simulink library "aerosimlib"  (Simulink 5.0)
values from neighbouring files (symbols this model uses):
  stdatm = [0 100 200 300 400 500 600 700 800 900 1000 1100 ... (4305 elements, 861x5)]    [stdatm.mat]
undefined symbols (not defined in the file or in its folder): AlphaBnd, b, BetaBnd, CDda, CDde, CDdf, CDdr, CDM, CDmin, CGempty, CGgross, CL0, CLa, CLalphadot, Clbeta, Clda, CLde, CLdf, Cldr, CLM, CLmind, Clp, CLq, Clr, Cm0, Cma, Cmalphadot, Cmde, Cmdf, CmM, Cmq, Cnbeta, Cnda, Cndr, Cnp, Cnr, CP, CT, CYbeta, CYda, CYdr, CYp, CYr, Displacement, dmy, Engine, EulerIni, FuelFlow, FuelIni, J, Jempty, Jeng, Jgross, Jprop, MAC, MAP, MAPLim, MassIni, MaxPower, mempty ... (+25)
libraries: aerosimlib x350, simulink3 x41
(part 2 of 10)

== system aerosimlib/Math ==
  2pi Bound : Subsystem
      mask Type: 2pi bound
      mask Description: Bounds the input angle to [0, 2pi]. When 0 bound is exceeded the output wraps back to 2pi; when the 2pi bound is exceeded the output wraps back to 0.
      mask Help:
      | Bounds the input angle to [0, 2pi]. When 0 bound is exceeded the output wraps back to 2pi; when the 2pi bound is exceeded the output wraps back to 0.
      | <P><B>Input:</B> any angle in radians, from -Inf to Inf;</P>
      | <P><B>Output:</B> an angle in radians between zero and 2pi.</P>
  Cross Product : Subsystem
      mask Type: Cross product
      mask Description: Computes the cross product of two vectors.
      mask Help:
      | The block computes the cross product of two three-dimensional vectors.
      | <P><B>Inputs:</B> two 3x1 vectors;</P>
      | <P><B>Output:</B> the 3x1 cross product vector.</P>
  Non-zero Sign : Subsystem
      mask Type: Non-zero sign
      mask Description: Sign function outputs 1 for input greater than or equal to 0, and -1 otherwise.
      mask Help: Sign function outputs 1 for input greater than or equal to 0, and -1 otherwise.
  Normalization : Subsystem
      mask Type: Vector normalization
      mask Description: Normalize a vector, e = v/|v|.
      mask Help:
      | The block normalizes the input vector.
      | <P><B>Input:</B> the nx1 vector;</P>
      | <P><B>Output:</B> the nx1 unit vector.</P>
  Vector norm : Subsystem
      mask Type: Vector norm-2
      mask Description: Compute the 2-norm (magnitude) of a vector, |v| = sqrt(v'v).
      mask Help:
      | The block compute the 2-norm (or magnitude) of a vector.
      | <P><B>Input:</B> nx1 vector;</P>
      | <P><B>Output:</B> scalar magnitude.</P>
  Zero Offset : Subsystem  mask(Zero offset){tol=10^-6}
      mask prompts: tol "Tolerance"
      mask help: This block outputs a value equal to the tolerance specified in the block parameters if the input falls within a sphere with this tolerance as radius and center in the origin. Otherwise, the output equals the input.
      mask Help: This block outputs a value equal to the tolerance specified in the block parameters if the input falls within a sphere with this tolerance as radius and center in the origin. Otherwise, the output equals the input.
  pi Bound : Subsystem
      mask Type: pi bound
      mask Description: Bounds the input angle to [-pi, pi]. When -pi bound is exceeded the output wraps back to pi; when the pi bound is exceeded the output wraps back to -pi.
      mask Help:
      | Bounds the input angle to [-pi, pi]. When -pi bound is exceeded the output wraps back to pi; when the pi bound is exceeded the output wraps back to -pi.
      | <P><B>Input:</B> any angle in radians, from -Inf to Inf;</P>
      | <P><B>Output:</B> an angle in radians between -pi and pi.</P>

== system aerosimlib/Pilot Interface ==
  CH F-16 Combat Stick : Subsystem  mask(CH F-16 Combat Stick){joyid=1, tsamp=0.02}
      mask prompts: joyid "Joystick ID:"; tsamp "Sample time:"
      mask help: Joystick interface for F-16 Combat Stick by CH Products.
      mask Help:
      | The block provides interface for the F-16 Combat Stick by CH Products.
      | <P><B>Outputs:</B>
      | <LI>Horiz axis = the current joystick position on the horizontal axis</LI>
      | <LI>Vert axis = the current joystick position on the vertical axis</LI>
      | <LI>Throttle axis = the current position of the throttle wheel</LI>
      | <LI>POV = the current state of the joystick hat switch (0=center, 1=up, -1=down, 2=right, -2=left)</LI>
      | <LI>Button 1-9 = the current states of the 9 available buttons</LI>
      | </P>
      | <P><B>Parameters:</B>
      | <LI>Joystick id = the identifier is used to differentiate between multiple joysticks, and it can be set to 1 or 2.</LI>
      | <LI>Sample time = the time interval at which the joystick data is sampled</LI>
      | </P>
  FS Interface : Subsystem  mask(FS interface){tsamp=0.2}
      mask prompts: tsamp "Sample time:"
      mask help: Microsoft Flight Simulator Interface that provides a visual output of the aircraft position and attitude.
      mask Help:
      | The block provides position and attitude information to Microsoft Flight Simulator for visual output of the aircraft behavior. The data transfer is based on Inter-Process Communication using FSUIPC module.
      | <P><B>Inputs:</B>
      | <LI> the 3x1 vector of geographic position;</LI>
      | <LI> the 3x1 vector of Euler angles;</LI>
      | <LI> scalar number representing airspeed.</LI></P>
  FlightGear Interface : Subsystem  mask(FlightGear 0.9.2 interface){hostname='localhost', port=5500, tsamp=0.02}
      mask prompts: hostname "Host name:"; tsamp "Sample time:"
      mask help:
      | FlightGear Flight Simulator Interface that provides a visual output of the aircraft position and attitude.
      | This driver can be used with FlightGear 0.9.2 only.
      mask Help:
      | The block provides position and attitude information to FlightGear Flight Simulator 0.9.2 for visual output of the aircraft behavior.
      | <P><B>Parameters:</B>
      | <LI>Sample time: the sample time at which data is sent to FlightGear;</LI>
      | <LI>Host name: the name or IP address of the machine on which FlightGear is running.</LI>
      | <LI>Port: the port number on the host machine.</LI>
      | </P>
      | <P><B>Inputs:</B>
      | <LI> the 3x1 vector of geographic position;</LI>
      | <LI> the 3x1 vector of Euler angles;</LI>
      | <LI> scalar number representing airspeed.</LI></P>
  FlightGear 0.9.4  Interface : Subsystem  mask(FlightGear 0.9.4 interface){hostname='localhost', port=5500, tsamp=0.02}
      mask prompts: hostname "Host name:"; tsamp "Sample time:"
      mask help:
      | FlightGear Flight Simulator Interface that provides a visual output of the aircraft position and attitude.
      | This driver can be used with FlightGear 0.9.4 only.
      mask Help:
      | The block provides position and attitude information to FlightGear Flight Simulator 0.9.4 for visual output of the aircraft behavior.
      | <P><B>Parameters:</B>
      | <LI>Sample time: the sample time at which data is sent to FlightGear;</LI>
      | <LI>Host name: the name or IP address of the machine on which FlightGear is running.</LI>
      | <LI>Port: the port number on the host machine.</LI>
      | </P>
      | <P><B>Inputs:</B>
      | <LI>Position =  the 3x1 vector of geographic position in [rad rad m];</LI>
      | <LI>Euler =  the 3x1 vector of Euler angles in radians;</LI>
      | <LI>Airspeed =  scalar number representing airspeed, in m/s;</LI>
      | <LI>VClimb = the climb rate, in m/s;</LI>
      | <LI>AGL = the altitude above ground, in meters;</LI>
      | <LI>VelNED = the 3x1 vector of groundspeed, in m/s;</LI>
      | <LI>Rates = the 3x1 vector of angular rates, in rad/s;</LI>
      | <LI>Acc = the 3x1 vector of body accelerations, in m/s^2;</LI>
      | <LI>Omega = the engine speed,in rad/s;</LI>
      | <LI>FuelFlow = the instananeous fuel flow, in grams per hour;</LI>
      | <LI>OutofFuel = set it to 1 to disable engine noise in FlightGear, otherwise set it to 0;</LI>
      | <LI>Controls = the 7x1 vector of aircraft controls [flap elevator aileron rudder throttle mixture ignition]; the first 4 aerodynamic controls should be normalized to [-1, 1].</LI>
      | </P>
  FlightGear 0.9.6  Interface : Subsystem  mask(FlightGear 0.9.6 interface){hostname='localhost', port=5500, tsamp=0.02}
      mask prompts: hostname "Host name:"; tsamp "Sample time:"
      mask help:
      | FlightGear Flight Simulator Interface that provides a visual output of the aircraft position and attitude.
      | This driver can be used with FlightGear 0.9.6 only.
      mask Help:
      | The block provides position and attitude information to FlightGear Flight Simulator 0.9.6 for visual output of the aircraft behavior.
      | <P><B>Parameters:</B>
      | <LI>Sample time: the sample time at which data is sent to FlightGear;</LI>
      | <LI>Host name: the name or IP address of the machine on which FlightGear is running.</LI>
      | <LI>Port: the port number on the host machine.</LI>
      | </P>
      | <P><B>Inputs:</B>
      | <LI>Position =  the 3x1 vector of geographic position in [rad rad m];</LI>
      | <LI>Euler =  the 3x1 vector of Euler angles in radians;</LI>
      | <LI>Airspeed =  scalar number representing airspeed, in m/s;</LI>
      | <LI>VClimb = the climb rate, in m/s;</LI>
      | <LI>AGL = the altitude above ground, in meters;</LI>
      | <LI>VelNED = the 3x1 vector of groundspeed, in m/s;</LI>
      | <LI>Rates = the 3x1 vector of angular rates, in rad/s;</LI>
      | <LI>Acc = the 3x1 vector of body accelerations, in m/s^2;</LI>
      | <LI>Omega = the engine speed,in rad/s;</LI>
      | <LI>FuelFlow = the instananeous fuel flow, in grams per hour;</LI>
      | <LI>OutofFuel = set it to 1 to disable engine noise in FlightGear, otherwise set it to 0;</LI>
      | <LI>Controls = the 7x1 vector of aircraft controls [flap elevator aileron rudder throttle mixture ignition]; the first 4 aerodynamic controls should be normalized to [-1, 1].</LI>
      | </P>
  FlightGear 0.9.8  Interface : Subsystem  mask(FlightGear 0.9.8 interface){hostname='localhost', port=5500, tsamp=0.02}
      mask prompts: hostname "Host name:"; tsamp "Sample time:"
      mask help:
      | FlightGear Flight Simulator Interface that provides a visual output of the aircraft position and attitude.
      | This driver can be used with FlightGear 0.9.8 only.
      mask Help:
      | The block provides position and attitude information to FlightGear Flight Simulator 0.9.8 for visual output of the aircraft behavior.
      | <P><B>Parameters:</B>
      | <LI>Sample time: the sample time at which data is sent to FlightGear;</LI>
      | <LI>Host name: the name or IP address of the machine on which FlightGear is running.</LI>
      | <LI>Port: the port number on the host machine.</LI>
      | </P>
      | <P><B>Inputs:</B>
      | <LI>Position =  the 3x1 vector of geographic position in [rad rad m];</LI>
      | <LI>Euler =  the 3x1 vector of Euler angles in radians;</LI>
      | <LI>Airspeed =  scalar number representing airspeed, in m/s;</LI>
      | <LI>VClimb = the climb rate, in m/s;</LI>
      | <LI>AGL = the altitude above ground, in meters;</LI>
      | <LI>VelNED = the 3x1 vector of groundspeed, in m/s;</LI>
      | <LI>Rates = the 3x1 vector of angular rates, in rad/s;</LI>
      | <LI>Acc = the 3x1 vector of body accelerations, in m/s^2;</LI>
      | <LI>Omega = the engine speed,in rad/s;</LI>
      | <LI>FuelFlow = the instananeous fuel flow, in grams per hour;</LI>
      | <LI>OutofFuel = set it to 1 to disable engine noise in FlightGear, otherwise set it to 0;</LI>
      | <LI>Controls = the 7x1 vector of aircraft controls [flap elevator aileron rudder throttle mixture ignition]; the first 4 aerodynamic controls should be normalized to [-1, 1].</LI>
      | </P>
  Joystick Interface : Subsystem  mask(Joystick interface){joyid=1, tsamp=0.02}
      mask prompts: joyid "Joystick ID:"; tsamp "Sample time:"
      mask help: Generic Windows joystick interface.
      mask Help:
      | The block provides a generic Windows joystick interface.
      | <P><B>Outputs:</B>
      | <LI>Axes = the 6x1 vector of current joystick position on the 6 available axes</LI>
      | <LI>Buttons = the 32x1 vector of current states of the 32 available buttons (0 or 1)</LI>
      | <LI>POV = the current state of the joystick hat switch (0=center, 1=up, -1=down, 2=right, -2=left)</LI>
      | </P>
      | <P><B>Parameters:</B>
      | <LI>Joystick ID = the identifier can be 1 or 2 and specifies which joystick to read, when the system has two joysticks installed.</LI>
      | <LI>Sample time = the time interval at which the joystick data is sampled</LI>
      | </P>
  R/C Transmitter  Interface : Subsystem  mask(R/C Transmitter Interface){joyid=1, tsamp=0.02}
      mask prompts: joyid "Joystick ID:"; tsamp "Sample time:"
      mask help: The R/C Transmitter Interface can be used with hardware devices that allow the use of R/C radios as Windows-compatible joysticks, such as the RealFlight Transmitter Interface and the Lew Engineering RCJOY.
      mask Help:
      | <P>The R/C Transmitter Interface can be used with hardware devices that allow the use of
      | R/C radios as Windows-compatible joysticks, such as the RealFlight Transmitter
      | Interface and the Lew Engineering RCJOY.</P>
      | <P><B>Outputs:</B>
      | <LI>Ch.1 Aileron = the Channel 1 output (usually aileron or roll cyclic on Futaba radios) normalized to [-1,1]</LI>
      | <LI>Ch.2 Elevator = the Channel 2 output (usually elevator or pitch cyclic on Futaba radios) normalized to [-1,1]</LI>
      | <LI>Ch.3 Throttle = the Channel 3 output (usually throttle/collective on Futaba radios) normalized to [0,1]</LI>
      | <LI>Ch.4 Rudder = the Channel 4 output (usually rudder or tail rotor on Futaba radios) normalize to [-1,1]]</LI>
      | <LI>Ch.5 Gear = the Channel 5 output (usually gear on Futaba radios), discrete 0 or 1</LI>
      | <LI>Ch.6 Flap = the Channel 6 output (usually flap on Futaba radios), discrete 0 or 1</LI>
      | <LI>Ch.7 Aux1 = the Channel 7 output (usually first auxiliary channel), discrete 0 or 1</LI>
      | <LI>Ch.8 Aux2 = the Channel 8 output (usually second auxiliary channel), discrete 0 or 1</LI>
      | </P>
      | <P><B>Parameters:</B>
      | <LI>Joystick id = the identifier is used to differentiate between multiple joysticks, and it can be set to 1 or 2.</LI>
      | <LI>Sample time = the time interval at which the joystick data is sampled</LI>
      | </P>

== system aerosimlib/Propulsion ==
  Fixed-pitch Propeller : Subsystem  mask(Fixed-pitch propeller model){J=J, CT=CT, CP=CP, R=Rprop}
      mask prompts: J "Advance ratio:"; CT "Coefficient of thrust:"; CP "Coefficient of power:"; R "Radius:"
      mask help: Fixed-pitch propeller model using look-up tables of thrust and power coefficients as functions of advance ratio.
      mask Help:
      | The block provides a fixed-pitch propeller model based on look-up tables for thrust and power coefficients as function of the advance ratio.
      | <P><B>Inputs:</B>
      | <LI>Airspeed = the current aircraft airspeed</LI>
      | <LI>rho = the air density at current aircraft altitude</LI>
      | <LI>Omega = the propeller rotation speed</LI>
      | </P>
      | <P><B>Output:</B>
      | <LI>Fprop = the thrust force generated by the propeller (on body x-axis)</LI>
      | <LI>Mprop = the moment generated by the propeller (on body x-axis)</LI>
      | <LI>PropCoeff = the 3x1 vector of propeller coefficients [J CT CP]</LI>
      | </P>
      | <P><B>Parameters:</B>
      | <LI>Advance ratio = the advance ratio vector for interpolation</LI>
      | <LI>Coefficient of thrust = the coefficient of thrust vector for interpolation</LI>
      | <LI>Coefficient of power = the coefficient of power vector for interpolation</LI>
      | <LI>Radius = the propeller radius</LI>
      | </P>
  GA Propulsion System : Subsystem  mask(General-aviation propulsion system){OmegaIni=OmegaIni, RPM=RPM, MAP=MAP, FuelFlow=FuelFlow, Power=Power, Jeng=Jeng, J=J, CT=CT, CP=CP, Rprop=Rprop, Jprop=Jprop, TSL=TSL}
      mask prompts: OmegaIni "Initial engine speed:"; RPM "Engine RPM vector:"; MAP "Engine MAP vector:"; FuelFlow "Engine fuel flow look-up table:"; Power "Engine power look-up table:"; Jeng "Engine moment of inertia:"; J "Propeller advance ratio vector:"; CT "Propeller coefficient of thrust vector:"; CP "Propeller coefficient of power vector:"; Rprop "Propeller radius:"; Jprop "Propeller moment of inertia:"; TSL "Sea-level temperature:"
      mask help: The block models a general aviation propulsion system including a piston engine and a fixed-pitch propeller.
      mask Help:
      | The block provides a general aviation propulsion system using the AeroSim piston engine and fixed-pitch propeller models.
      | <P><B>Inputs:</B>
      | <LI>Control = the 3x1 engine control vector [Throttle Mixture Ignition]</LI>
      | <LI>OutofFuel = the out-of-fuel flag (0 or 1)</LI>
      | <LI>p = the static pressure at current altitude, in Pa</LI>
      | <LI>T = the air temperature at current altitude, in K</LI>
      | <LI>rho = the air density at current altitude, in kg/m^3</LI>
      | <LI>WindAxesVel = the 3x1 vector of body velocities in wind axes [Airspeed Sideslip Angle-of-attack] in [m/s rad rad]</LI>
      | <LI>RST = the integrator reset flag (rising edge)</LI>
      | </P>
      | <P><B>Output:</B>
      | <LI>Fprop = the 3x1 vector of propulsion system forces applied to the airframe, at the propeller hub location</LI>
      | <LI>Mprop = the 3x1 vector of propulsion system moments applied to the airframe</LI>
      | <LI>Omega = the engine shaft rotation speed, in rad/s</LI>
      | <LI>FuelFlow = the mass fuel flow, in kg/s</LI>
      | <LI>EngCoeff = the 5x1 engine coefficient vector [MAP Airflow Fuelflow BSFC Power] in [kPa kg/s kg/s g/(W*hr) W]</LI>
      | <LI>PropCoeff = the 3x1 propeller coefficient vector [J CT CP]</LI>
      | </P>
      | <P><B>Parameters:</B>
      | <LI>Initial engine speed = the initial value for the engine speed, in rad/s</LI>
      | <LI>RPM vector = the engine speed interpolation vector, in rpm</LI>
      | <LI>MAP vector = the manifold air pressure interpolation vector, in kPa</LI>
      | <LI>Fuel flow = the 2-D look-up table for fuel flow, as function of MAP and RPM, in g/hr</LI>
      | <LI>Power = the 2-D look-up table for power, as function of MAP and RPM, in W</LI>
      | <LI>Engine moment of inertia = the moment of inertia of the rotating engine parts (shaft)</LI>
      | <LI>Advance ratio = the advance ratio vector for interpolation</LI>
      | <LI>Coefficient of thrust = the coefficient of thrust vector for interpolation</LI>
      | <LI>Coefficient of power = the coefficient of power vector for interpolation</LI>
      | <LI>Radius = the propeller radius</LI>
      | <LI>Propeller moment of inertia = the moment of inertia of the propeller</LI>
      | <LI>Sea-level temperature = the ambient temperature for which the above engine look-up tables are given</LI>
      | </P>
  Piston Engine : Subsystem  mask(Piston Engine){RPM=RPM, MAP=MAP, fflow=FuelFlow, Power=Power, TSL=TSL}
      mask prompts: RPM "RPM vector:"; MAP "MAP vector:"; fflow "Fuel flow 2-D look-up table:"; Power "Power 2-D look-up table:"; TSL "Sea-level temperature:"
      mask help: The piston engine model computes the engine parameters at current throttle setting, engine rpm, and altitude.
      mask Help:
      | The block provides a piston engine model based on look-up tables for manifold pressure, engine speed (rpm), fuel flow and power.
      | <P><B>Inputs:</B>
      | <LI>Thr = the throttle command (as a fraction of atmospheric pressure)</LI>
      | <LI>Mix = the air to fuel mixture ratio</LI>
      | <LI>Omega = the engine shaft rotation speed</LI>
      | <LI>p = the atmospheric pressure, in Pa</LI>
      | <LI>T = the atmospheric temperature, in K</LI>
      | </P>
      | <P><B>Output:</B>
      | <LI>MAP = the manifold air pressure, in kPa</LI>
      | <LI>AirFlow = the mass air flow, in kg/s</LI>
      | <LI>FuelFlow = the mass fuel flow, in kg/s</LI>
      | <LI>BSFC = the brake-specific fuel consumption, in g/(W*hr)</LI>
      | <LI>Power = the engine power, in W</LI>
      | <LI>Torque = the engine shaft torque, in N*m</LI>
      | </P>
      | <P><B>Parameters:</B>
      | <LI>RPM vector = the engine speed interpolation vector, in rpm</LI>
      | <LI>MAP vector = the manifold air pressure interpolation vector, in kPa</LI>
      | <LI>Fuel flow = the 2-D look-up table for fuel flow, as function of MAP and RPM, in g/hr</LI>
      | <LI>Power = the 2-D look-up table for power, as function of MAP and RPM, in W</LI>
      | <LI>Sea-level temperature = the ambient temperature for which the above engine look-up tables are given</LI>
      | </P>

== system aerosimlib/Sensors ==
  Analog Sensors : Subsystem
  Digital Sensors : Subsystem
  Generic Sensors : Subsystem
  Noise Correlation : Subsystem

== system aerosimlib/Transformations ==
  Body-Inertial DCM From Euler Angles : Subsystem
      mask Type: Body-Inertial DCM
      mask Description: Compute the direction cosine matrix required for inertial-to-body frame transformation.
      mask Help:
      | The block computes the Direction Cosine matrix which is the rotation matrix from inertial to body frame, given the vehicle attitude in Euler angles.
      | <P><B>Input:</B> the 3x1 vector of Euler angles;</P>
      | <P><B>Output:</B> the 3x3 Direction Cosine matrix.</P>
  Body-Inertial DCM From Quaternions : Subsystem
      mask Type: Body-Inertial DCM
      mask Description: Compute the direction cosine matrix required for inertial-to-body frame transformation.
      mask Help:
      | The block computes the Direction Cosine matrix which is the rotation matrix from inertial to body frame, given the Euler-Rodrigues quaternions.
      | <P><B>Input:</B> the 4x1 vector of quaterions;</P>
      | <P><B>Output:</B> the 3x3 Direction Cosine matrix.</P>
  Body-Wind DCM : Subsystem
      mask Type: Body-Wind DCM
      mask Description: Compute the body-axes to wind-axes direction cosine matrix.
      mask Help:
      | The block computes the Direction Cosine matrix that defines the rotation from body to wind axes, given the sideslip angle and the angle-of-attack.
      | <P><B>Input:</B> the 3x1 vector of wind axes velocity components (airspeed, sideslip, angle-of-attack);</P>
      | <P><B>Output:</B> the 3x3 Direction Cosine matrix.</P>
  Body2LTP : Subsystem
      mask Type: Body to LTP
      mask Description: Fast frame transformation from body to local tangential plane (rotation by phi and theta).
  ECEF Position : Subsystem
      mask Type: ECEF Position
      mask Description: Compute ECEF (Earth-centered Earth-fixed) position from LLA (Latitude, Longitude, Altitude) position.
      mask Help:
      | The block computes the coordinates of the vehicle in the Earth-Centered Earth-Fixed frame, given the coordinates in geographic frame and local Earth radii.
      | <P><B>Inputs:</B>
      | <LI>LLA = the 3x1 position vector (Latitude, Longitude, Altitude);</LI>
      | <LI>Rmeridian = local meridian radius of the Earth;</LI>
      | <LI>Rnormal = local normal radius of the Earth;</LI></P>
      | <P><B>Output:</B> the 3x1 vector of ECEF position (X, Y, Z).</P>
  Euler Angles From Quaternions : Subsystem
      mask Type: Euler Angles
      mask Description: Compute Euler angles from Euler-Rodrigues quaternions.
      mask Help:
      | The block computes the three Euler angles (roll, pitch, heading) of the vehicle based on the Euler-Rodrigues quaternions.
      | <P><B>Input:</B> the 4x1 vector of quaternions;</P>
      | <P><B>Output:</B> the 3x1 vector of Euler angles.</P>
  Euler Angles  From DCM : Subsystem
      mask Type: Euler angles from DCM
      mask Description: Compute Euler angles given the Direction Cosine Matrix.
      mask Help:
      | The block extracts the 3 Euler angles (roll, pitch, and heading) from elements of the Direction Cosine matrix.
      | <P><B>Input:</B> a 3x3 Direction Cosine matrix;</P>
      | <P><B>Output:</B> a 3x1 vector with the Euler angles.</P>
  LTP2Body : Subsystem
      mask Type: LTP to Body
      mask Description: Fast frame transformation from local tangential plane to body frame (rotation by phi and theta).
  Quaternions From Euler Angles : Subsystem
      mask Type: Quaternions
      mask Description: Compute quaternions from Euler angles.
      mask Help:
      | The block computes the four quaternions (q0, qx, qy, qz) of the vehicle based on the Euler angles.
      | <P><B>Input:</B> the 3x1 vector of Euler angles.</P>
      | <P><B>Output:</B> the 4x1 vector of quaternions;</P>

== system aerosimlib/Unit Conversion ==
  Angular position : Subsystem
  Angular velocity : Subsystem
  Distance : Subsystem
  Force : Subsystem
  Mass : Subsystem
  Pressure : Subsystem
  Temperature : Subsystem
  Velocity : Subsystem
  Volume : Subsystem

== system aerosimlib/Actuators/D/A Converter ==
  Digital : Inport
  Count size in Volts : Product  Inputs=*/  SaturateOnIntegerOverflow=on  InputSameDT=on
  Max Counts : Constant  Value=2^Bits
  Max Volts : Constant  Value=MaxVolts
  Min Volts : Constant  Value=MinVolts
  Saturation : Saturate  UpperLimit=MaxVolts  LowerLimit=MinVolts
  Sum : Sum  Inputs=|+-  SaturateOnIntegerOverflow=on  InputSameDT=on
  Voltage : Product  SaturateOnIntegerOverflow=on  InputSameDT=on
  Analog : Outport
  wires:
  Digital/1 -> Voltage/1
  Voltage/1 -> Saturation/1
  Max Volts/1 -> Sum/1
  Min Volts/1 -> Sum/2
  Max Counts/1 -> Count size in Volts/2
  Sum/1 -> Count size in Volts/1
  Count size in Volts/1 -> Voltage/2
  Saturation/1 -> Analog/1

== system aerosimlib/Actuators/Simple Actuator (1st-order dynamics) ==
  Input : Inport  PortDimensions=1
  Look-Up Table : Lookup  InputValues=[MinCounts MaxCounts]  OutputValues=[MinAct MaxAct]  SaturateOnIntegerOverflow=on
  Rate Limiter : RateLimiter  RisingSlewLimit=MaxRate  FallingSlewLimit=-MaxRate
  Saturation : Saturate  UpperLimit=MaxCounts  LowerLimit=MinCounts
  Transfer Fcn : TransferFcn  Denominator=[Lag 1]
  Output : Outport
  wires:
  Transfer Fcn/1 -> Output/1
  Rate Limiter/1 -> Transfer Fcn/1
  Saturation/1 -> Look-Up Table/1
  Input/1 -> Saturation/1
  Look-Up Table/1 -> Rate Limiter/1

== system aerosimlib/Actuators/Simple Actuator (2nd-order dynamics) ==
  Input : Inport  PortDimensions=1
  Look-Up Table : Lookup  InputValues=[MinCounts MaxCounts]  OutputValues=[MinAct MaxAct]  SaturateOnIntegerOverflow=on
  Rate Limiter : RateLimiter  RisingSlewLimit=MaxRate  FallingSlewLimit=-MaxRate
  Saturation : Saturate  UpperLimit=MaxCounts  LowerLimit=MinCounts
  Transfer Fcn : TransferFcn  Numerator=[wn^2]  Denominator=[1 2*zeta*wn wn^2]
  Output : Outport
  wires:
  Look-Up Table/1 -> Rate Limiter/1
  Input/1 -> Saturation/1
  Saturation/1 -> Look-Up Table/1
  Rate Limiter/1 -> Transfer Fcn/1
  Transfer Fcn/1 -> Output/1

== system aerosimlib/Aerodynamics/Aerodynamic Force ==
  note: Get aerodynamic forces in
      | wind axes
  note: Get aerodynamic forces
      | in body axes
  CD : Inport  PortDimensions=1
  CY : Inport  Port=2  PortDimensions=1
  CL : Inport  Port=3  PortDimensions=1
  pdyn : Inport  Port=4  PortDimensions=1
  WindAxesVel : Inport  Port=5  PortDimensions=[3 1]
  Body-Wind DCM : aerosimlib/Transformations/Body-Wind DCM
  ChSign : Gain  Gain=-1  SaturateOnIntegerOverflow=on
  ChSign1 : Gain  Gain=-1  SaturateOnIntegerOverflow=on
  DCM' : Math  Operator=transpose
  Mux : Mux  Inputs=3
  Product : Product  Inputs=3  SaturateOnIntegerOverflow=on  InputSameDT=on
  Product1 : Product  Multiplication=Matrix(*)  SaturateOnIntegerOverflow=on  InputSameDT=on
  Wing area : Constant  Value=S
  Faero : Outport
  wires:
  ChSign1/1 -> Mux/3
  ChSign/1 -> Mux/1
  CD/1 -> ChSign/1
  CY/1 -> Mux/2
  CL/1 -> ChSign1/1
  Mux/1 -> Product/1
  pdyn/1 -> Product/2
  Wing area/1 -> Product/3
  WindAxesVel/1 -> Body-Wind DCM/1
  DCM'/1 -> Product1/1
  Body-Wind DCM/1 -> DCM'/1
  Product/1 -> Product1/2
  Product1/1 -> Faero/1

== system aerosimlib/Aerodynamics/Aerodynamic Moment ==
  note: Sources
  note: Compute moments
  note: Output
  Cl : Inport  PortDimensions=1
  Cm : Inport  Port=2  PortDimensions=1
  Cn : Inport  Port=3  PortDimensions=1
  pdyn : Inport  Port=4  PortDimensions=1
  Mux : Mux  Inputs=3
  Pitch : Product  Inputs=4  SaturateOnIntegerOverflow=on  InputSameDT=on
  Roll : Product  Inputs=4  SaturateOnIntegerOverflow=on  InputSameDT=on
  Wing area : Constant  Value=S
  Wing chord : Constant  Value=c
  Wing span : Constant  Value=b
  Yaw : Product  Inputs=4  SaturateOnIntegerOverflow=on  InputSameDT=on
  Maero : Outport
  wires:
  Cl/1 -> Roll/4
  Cm/1 -> Pitch/4
  Cn/1 -> Yaw/4
  pdyn/1 -> Roll/1, Pitch/1, Yaw/1
  Wing area/1 -> Roll/2, Pitch/2, Yaw/2
  Wing chord/1 -> Pitch/3
  Wing span/1 -> Roll/3, Yaw/3
  Roll/1 -> Mux/1
  Mux/1 -> Maero/1
  Pitch/1 -> Mux/2
  Yaw/1 -> Mux/3

== system aerosimlib/Aerodynamics/Drag Coefficient ==
  note: Drag component build-up
  note: Sources
  WindAxesVel : Inport  PortDimensions=[3 1]
  Control : Inport  Port=2  PortDimensions=[4 1]
  CL : Inport  Port=3  PortDimensions=1
  Mach : Inport  Port=4  PortDimensions=1
  Abs{,1..3} (4 alike) : Abs  SaturateOnIntegerOverflow=on
  CD0 : Constant  Value=CD0
  CDM : Gain  Gain=CDM  SaturateOnIntegerOverflow=on
  CDda : Gain  Gain=CDda  SaturateOnIntegerOverflow=on
  CDde : Gain  Gain=CDde  SaturateOnIntegerOverflow=on
  CDdf : Gain  Gain=CDdf  SaturateOnIntegerOverflow=on
  CDdr : Gain  Gain=CDdr  SaturateOnIntegerOverflow=on
  CL min drag : Constant  Value=CL0
  CL^2 : Math  Operator=square
  Demux : Demux
  Demux1 : Demux  Outputs=3
  Induced Drag : Gain  Gain=k  SaturateOnIntegerOverflow=on
  Sum : Sum  Inputs=|+-  SaturateOnIntegerOverflow=on  InputSameDT=on
  Sum2 : Sum  Inputs=+++++++  SaturateOnIntegerOverflow=on  InputSameDT=on
  Terminator : Terminator
  Terminator1 : Terminator
  Terminator2 : Terminator
  CD : Outport
  wires:
  CDM/1 -> Sum2/7
  Mach/1 -> CDM/1
  CL min drag/1 -> Sum/2
  CL/1 -> Sum/1
  Sum/1 -> CL^2/1
  Sum2/1 -> CD/1
  CDdr/1 -> Abs3/1
  CDda/1 -> Abs2/1
  CDde/1 -> Abs1/1
  CDdf/1 -> Abs/1
  Induced Drag/1 -> Sum2/2
  CD0/1 -> Sum2/1
  CL^2/1 -> Induced Drag/1
  Control/1 -> Demux/1
  Demux/4 -> CDdr/1
  Demux/3 -> CDda/1
  Demux/2 -> CDde/1
  Demux/1 -> CDdf/1
  WindAxesVel/1 -> Demux1/1
  Abs/1 -> Sum2/3
  Abs1/1 -> Sum2/4
  Abs2/1 -> Sum2/5
  Abs3/1 -> Sum2/6
  Demux1/1 -> Terminator/1
  Demux1/2 -> Terminator1/1
  Demux1/3 -> Terminator2/1

== system aerosimlib/Aerodynamics/Dynamic Pressure ==
  WindAxesVel : Inport  PortDimensions=[3 1]
  rho : Inport  Port=2  PortDimensions=1
  0.5*rho*Va^2 : Product  SaturateOnIntegerOverflow=on  InputSameDT=on
  Demux : Demux  Outputs=3
  Gain : Gain  Gain=1/2  SaturateOnIntegerOverflow=on
  Terminator : Terminator
  Terminator1 : Terminator
  Va^2 : Math  Operator=square
  pdyn : Outport
  wires:
  rho/1 -> Gain/1
  Demux/3 -> Terminator1/1
  Demux/2 -> Terminator/1
  Demux/1 -> Va^2/1
  WindAxesVel/1 -> Demux/1
  Va^2/1 -> 0.5*rho*Va^2/1
  Gain/1 -> 0.5*rho*Va^2/2
  0.5*rho*Va^2/1 -> pdyn/1

== system aerosimlib/Aerodynamics/Lift Coefficient ==
  note: Lift component build-up
  note: Sources
  WindAxesVel : Inport  PortDimensions=[3 1]
  Control : Inport  Port=2  PortDimensions=[4 1]
  AlphaBetaDot : Inport  Port=3  PortDimensions=[2 1]
  AngularRates : Inport  Port=4  PortDimensions=[3 1]
  Mach : Inport  Port=5  PortDimensions=1
  2 : Gain  Gain=2  SaturateOnIntegerOverflow=on
  CL*c/(2V) : Product  Inputs=**/  SaturateOnIntegerOverflow=on  InputSameDT=on
  CL0 : Constant  Value=CL0
  CLM : Gain  Gain=CLM  SaturateOnIntegerOverflow=on
  CLalpha : Gain  Gain=CLalpha  SaturateOnIntegerOverflow=on
  CLalphadot : Gain  Gain=CLalphadot  SaturateOnIntegerOverflow=on
  CLde : Gain  Gain=CLde  SaturateOnIntegerOverflow=on
  CLdf : Gain  Gain=CLdf  SaturateOnIntegerOverflow=on
  CLq : Gain  Gain=CLq  SaturateOnIntegerOverflow=on
  Demux : Demux
  Demux1 : Demux  Outputs=3
  Demux2 : Demux  Outputs=2
  Demux3 : Demux  Outputs=3
  Sum : Sum  SaturateOnIntegerOverflow=on  InputSameDT=on
  Sum2 : Sum  Inputs=++++++  SaturateOnIntegerOverflow=on  InputSameDT=on
  Terminator{,1..5} (6 alike) : Terminator
  Wing chord : Constant  Value=c
  CL : Outport
  wires:
  CLM/1 -> Sum2/6
  Mach/1 -> CLM/1
  Demux3/3 -> Terminator5/1
  Demux3/2 -> CLq/1
  Demux3/1 -> Terminator4/1
  AngularRates/1 -> Demux3/1
  Sum2/1 -> CL/1
  CL*c/(2V)/1 -> Sum2/5
  CLde/1 -> Sum2/4
  CLdf/1 -> Sum2/3
  CLalpha/1 -> Sum2/2
  CL0/1 -> Sum2/1
  Sum/1 -> CL*c/(2V)/1
  CLalphadot/1 -> Sum/1
  AlphaBetaDot/1 -> Demux2/1
  Demux2/2 -> Terminator3/1
  Demux2/1 -> CLalphadot/1
  Control/1 -> Demux/1
  Demux/4 -> Terminator2/1
  Demux/3 -> Terminator1/1
  Demux/2 -> CLde/1
  Demux/1 -> CLdf/1
  Demux1/3 -> CLalpha/1
  Demux1/2 -> Terminator/1
  Demux1/1 -> 2/1
  CLq/1 -> Sum/2
  Wing chord/1 -> CL*c/(2V)/2
  2/1 -> CL*c/(2V)/3
  WindAxesVel/1 -> Demux1/1

== system aerosimlib/Aerodynamics/Pitch Moment Coefficient ==
  note: Pitch moment component build-up
  note: Sources
  WindAxesVel : Inport  PortDimensions=[3 1]
  Control : Inport  Port=2  PortDimensions=[4 1]
  AlphaBetaDot : Inport  Port=3  PortDimensions=[2 1]
  AngularRates : Inport  Port=4  PortDimensions=[3 1]
  Mach : Inport  Port=5  PortDimensions=1
  2 : Gain  Gain=2  SaturateOnIntegerOverflow=on
  Cm*c/(2V) : Product  Inputs=**/  SaturateOnIntegerOverflow=on  InputSameDT=on
  Cm0 : Constant  Value=Cm0
  CmM : Gain  Gain=CmM  SaturateOnIntegerOverflow=on
  Cmalpha : Gain  Gain=Cma  SaturateOnIntegerOverflow=on
  Cmalphadot : Gain  Gain=Cmalphadot  SaturateOnIntegerOverflow=on
  Cmde : Gain  Gain=Cmde  SaturateOnIntegerOverflow=on
  Cmdf : Gain  Gain=Cmdf  SaturateOnIntegerOverflow=on
  Cmq : Gain  Gain=Cmq  SaturateOnIntegerOverflow=on
  Demux : Demux
  Demux1 : Demux  Outputs=3
  Demux2 : Demux  Outputs=2
  Demux3 : Demux  Outputs=3
  Sum : Sum  SaturateOnIntegerOverflow=on  InputSameDT=on
  Sum2 : Sum  Inputs=++++++  SaturateOnIntegerOverflow=on  InputSameDT=on
  Terminator{,1..5} (6 alike) : Terminator
  Wing chord : Constant  Value=c
  Cm : Outport
  wires:
  CmM/1 -> Sum2/6
  Sum2/1 -> Cm/1
  Cm*c/(2V)/1 -> Sum2/5
  Cmde/1 -> Sum2/4
  Cmdf/1 -> Sum2/3
  Cmalpha/1 -> Sum2/2
  Cm0/1 -> Sum2/1
  Sum/1 -> Cm*c/(2V)/1
  Cmalphadot/1 -> Sum/1
  Cmq/1 -> Sum/2
  Wing chord/1 -> Cm*c/(2V)/2
  2/1 -> Cm*c/(2V)/3
  Mach/1 -> CmM/1
  Demux3/3 -> Terminator5/1
  Demux3/2 -> Cmq/1
  Demux3/1 -> Terminator4/1
  AngularRates/1 -> Demux3/1
  AlphaBetaDot/1 -> Demux2/1
  Demux2/2 -> Terminator3/1
  Demux2/1 -> Cmalphadot/1
  Control/1 -> Demux/1
  Demux/4 -> Terminator2/1
  Demux/3 -> Terminator1/1
  Demux/2 -> Cmde/1
  Demux/1 -> Cmdf/1
  Demux1/3 -> Cmalpha/1
  Demux1/2 -> Terminator/1
  Demux1/1 -> 2/1
  WindAxesVel/1 -> Demux1/1

== system aerosimlib/Aerodynamics/Roll Moment Coefficient ==
  note: Roll moment component build-up
  note: Sources
  WindAxesVel : Inport  PortDimensions=[3 1]
  Control : Inport  Port=2  PortDimensions=[4 1]
  AngularRates : Inport  Port=3  PortDimensions=[3 1]
  2 : Gain  Gain=2  SaturateOnIntegerOverflow=on
  Cl*b/(2V) : Product  Inputs=**/  SaturateOnIntegerOverflow=on  InputSameDT=on
  Clbeta : Gain  Gain=Clbeta  SaturateOnIntegerOverflow=on
  Clda : Gain  Gain=Clda  SaturateOnIntegerOverflow=on
  Cldr : Gain  Gain=Cldr  SaturateOnIntegerOverflow=on
  Clp : Gain  Gain=Clp  SaturateOnIntegerOverflow=on
  Clr : Gain  Gain=Clr  SaturateOnIntegerOverflow=on
  Demux : Demux
  Demux1 : Demux  Outputs=3
  Demux3 : Demux  Outputs=3
  Sum : Sum  SaturateOnIntegerOverflow=on  InputSameDT=on
  Sum2 : Sum  Inputs=++++  SaturateOnIntegerOverflow=on  InputSameDT=on
  Terminator{,1..3} (4 alike) : Terminator
  Wing span : Constant  Value=b
  Cl : Outport
  wires:
  Sum2/1 -> Cl/1
  Cl*b/(2V)/1 -> Sum2/4
  Cldr/1 -> Sum2/3
  Clda/1 -> Sum2/2
  Clbeta/1 -> Sum2/1
  Demux3/3 -> Clr/1
  Demux3/2 -> Terminator3/1
  Demux3/1 -> Clp/1
  AngularRates/1 -> Demux3/1
  Control/1 -> Demux/1
  Demux/4 -> Cldr/1
  Demux/3 -> Clda/1
  Demux/2 -> Terminator2/1
  Demux/1 -> Terminator1/1
  Demux1/3 -> Terminator/1
  Demux1/2 -> Clbeta/1
  Demux1/1 -> 2/1
  WindAxesVel/1 -> Demux1/1
  2/1 -> Cl*b/(2V)/3
  Wing span/1 -> Cl*b/(2V)/2
  Sum/1 -> Cl*b/(2V)/1
  Clr/1 -> Sum/2
  Clp/1 -> Sum/1

== system aerosimlib/Aerodynamics/Side Force Coefficient ==
  note: Side force coefficient component build-up
  note: Sources
  WindAxesVel : Inport  PortDimensions=[3 1]
  Control : Inport  Port=2  PortDimensions=[4 1]
  AngularRates : Inport  Port=3  PortDimensions=[3 1]
  2 : Gain  Gain=2  SaturateOnIntegerOverflow=on
  CY*b/(2V) : Product  Inputs=**/  SaturateOnIntegerOverflow=on  InputSameDT=on
  CYbeta : Gain  Gain=CYbeta  SaturateOnIntegerOverflow=on
  CYda : Gain  Gain=CYda  SaturateOnIntegerOverflow=on
  CYdr : Gain  Gain=CYdr  SaturateOnIntegerOverflow=on
  CYp : Gain  Gain=CYp  SaturateOnIntegerOverflow=on
  CYr : Gain  Gain=CYr  SaturateOnIntegerOverflow=on
  Demux : Demux
  Demux1 : Demux  Outputs=3
  Demux3 : Demux  Outputs=3
  Sum : Sum  SaturateOnIntegerOverflow=on  InputSameDT=on
  Sum2 : Sum  Inputs=++++  SaturateOnIntegerOverflow=on  InputSameDT=on
  Terminator{,1..3} (4 alike) : Terminator
  Wing span : Constant  Value=b
  CY : Outport
  wires:
  Sum2/1 -> CY/1
  CY*b/(2V)/1 -> Sum2/4
  CYdr/1 -> Sum2/3
  CYda/1 -> Sum2/2
  CYbeta/1 -> Sum2/1
  Demux3/3 -> CYr/1
  Demux3/2 -> Terminator3/1
  Demux3/1 -> CYp/1
  AngularRates/1 -> Demux3/1
  Control/1 -> Demux/1
  Demux/4 -> CYdr/1
  Demux/3 -> CYda/1
  Demux/2 -> Terminator2/1
  Demux/1 -> Terminator1/1
  Demux1/3 -> Terminator/1
  Demux1/2 -> CYbeta/1
  Demux1/1 -> 2/1
  WindAxesVel/1 -> Demux1/1
  2/1 -> CY*b/(2V)/3
  Wing span/1 -> CY*b/(2V)/2
  Sum/1 -> CY*b/(2V)/1
  CYr/1 -> Sum/2
  CYp/1 -> Sum/1

== system aerosimlib/Aerodynamics/Wind-axes Velocities ==
  note: Sources
  note: Get airspeed
  note: Get angle-of-attack
  note: Get sideslip
  note: Output
  Vbody : Inport  PortDimensions=[3 1]
  Wbody : Inport  Port=2  PortDimensions=[3 1]
  SoundSpd : Inport  Port=3  PortDimensions=1
  AOA Saturation : Saturate  UpperLimit=alphabnd(2)  LowerLimit=alphabnd(1)
  Airspeed Saturation : Saturate  UpperLimit=Vabnd(2)  LowerLimit=Vabnd(1)
  Demux : Demux  Outputs=3
  Derivative : Derivative
  Mux : Mux  Inputs=3
  Mux1 : Mux  Inputs=2
  Sideslip Saturation : Saturate  UpperLimit=betabnd(2)  LowerLimit=betabnd(1)
  Sum : Sum  Inputs=|+-  SaturateOnIntegerOverflow=on  InputSameDT=on
  Trigonometric Function : Trigonometry  Operator=atan
  Trigonometric Function1 : Trigonometry  Operator=asin
  V/a : Product  Inputs=*/  SaturateOnIntegerOverflow=on  InputSameDT=on
  Vector norm : aerosimlib/Math/Vector norm
  Zero Offset : aerosimlib/Math/Zero Offset  tol=10^-6
  Zero Offset1 : aerosimlib/Math/Zero Offset  tol=10^-6
  v/Va : Product  Inputs=*/  SaturateOnIntegerOverflow=on  InputSameDT=on
  w/u : Product  Inputs=*/  SaturateOnIntegerOverflow=on  InputSameDT=on
  WindAxesVel : Outport
  AlphaBetaDot : Outport  Port=2
  Mach : Outport  Port=3
  wires:
  AOA Saturation/1 -> Mux/3
  Sideslip Saturation/1 -> Mux/2
  Airspeed Saturation/1 -> Mux/1
  V/a/1 -> Mach/1
  SoundSpd/1 -> V/a/2
  Derivative/1 -> AlphaBetaDot/1
  Mux1/1 -> Derivative/1
  Vbody/1 -> Sum/1
  Wbody/1 -> Sum/2
  Sum/1 -> Demux/1, Vector norm/1
  Demux/1 -> Zero Offset/1
  Demux/2 -> v/Va/1
  Demux/3 -> w/u/1
  Vector norm/1 -> Airspeed Saturation/1, V/a/1, Zero Offset1/1
  w/u/1 -> Trigonometric Function/1
  Trigonometric Function/1 -> AOA Saturation/1, Mux1/1
  v/Va/1 -> Trigonometric Function1/1
  Trigonometric Function1/1 -> Sideslip Saturation/1, Mux1/2
  Mux/1 -> WindAxesVel/1
  Zero Offset/1 -> w/u/2
  Zero Offset1/1 -> v/Va/2

== system aerosimlib/Aerodynamics/Yaw Moment Coefficient ==
  note: Sources
  note: Rol moment component build-up
  WindAxesVel : Inport  PortDimensions=[3 1]
  Control : Inport  Port=2  PortDimensions=[4 1]
  AngularRates : Inport  Port=3  PortDimensions=[3 1]
  2 : Gain  Gain=2  SaturateOnIntegerOverflow=on
  Cn*b/(2V) : Product  Inputs=**/  SaturateOnIntegerOverflow=on  InputSameDT=on
  Cnbeta : Gain  Gain=Cnbeta  SaturateOnIntegerOverflow=on
  Cnda : Gain  Gain=Cnda  SaturateOnIntegerOverflow=on
  Cndr : Gain  Gain=Cndr  SaturateOnIntegerOverflow=on
  Cnp : Gain  Gain=Cnp  SaturateOnIntegerOverflow=on
  Cnr : Gain  Gain=Cnr  SaturateOnIntegerOverflow=on
  Demux : Demux
  Demux1 : Demux  Outputs=3
  Demux3 : Demux  Outputs=3
  Sum : Sum  SaturateOnIntegerOverflow=on  InputSameDT=on
  Sum2 : Sum  Inputs=++++  SaturateOnIntegerOverflow=on  InputSameDT=on
  Terminator{,1..3} (4 alike) : Terminator
  Wing span : Constant  Value=b
  Cn : Outport
  wires:
  Cnp/1 -> Sum/1
  Cnr/1 -> Sum/2
  Sum/1 -> Cn*b/(2V)/1
  Wing span/1 -> Cn*b/(2V)/2
  2/1 -> Cn*b/(2V)/3
  WindAxesVel/1 -> Demux1/1
  Demux1/1 -> 2/1
  Demux1/2 -> Cnbeta/1
  Demux1/3 -> Terminator/1
  Demux/1 -> Terminator1/1
  Demux/2 -> Terminator2/1
  Demux/3 -> Cnda/1
  Demux/4 -> Cndr/1
  Control/1 -> Demux/1
  AngularRates/1 -> Demux3/1
  Demux3/1 -> Cnp/1
  Demux3/2 -> Terminator3/1
  Demux3/3 -> Cnr/1
  Cnbeta/1 -> Sum2/1
  Cnda/1 -> Sum2/2
  Cndr/1 -> Sum2/3
  Cn*b/(2V)/1 -> Sum2/4
  Sum2/1 -> Cn/1

== system aerosimlib/Atmosphere/Background Wind ==
  note: Wind speed in body axes
  WindsNED : Inport  PortDimensions=[3 1]
  DCM : Inport  Port=2  PortDimensions=[3 3]
  Derivative : Derivative
  Product : Product  Multiplication=Matrix(*)  SaturateOnIntegerOverflow=on  InputSameDT=on
  Product1 : Product  Multiplication=Matrix(*)  SaturateOnIntegerOverflow=on  InputSameDT=on
  WindVel : Outport
  WindAcc : Outport  Port=2
  wires:
  Product1/1 -> WindAcc/1
  Derivative/1 -> Product1/2
  Product/1 -> WindVel/1
  WindsNED/1 -> Derivative/1, Product/2
  DCM/1 -> Product1/1, Product/1

== system aerosimlib/Atmosphere/Standard Atmosphere ==
  note: 1976 Standard Atmosphere Look-up Tables
  note: Outputs
  note: Sources
  MSLAlt : Inport  PortDimensions=1
  Density LUT : Lookup  InputValues=stdatm(:,1)  OutputValues=stdatm(:,4)  SaturateOnIntegerOverflow=on
  Pressure LUT : Lookup  InputValues=stdatm(:,1)  OutputValues=stdatm(:,3)  SaturateOnIntegerOverflow=on
  Saturation : Saturate  UpperLimit=86000  LowerLimit=0
  Speed of sound  LUT : Lookup  InputValues=stdatm(:,1)  OutputValues=stdatm(:,5)  SaturateOnIntegerOverflow=on
  Temperature LUT : Lookup  InputValues=stdatm(:,1)  OutputValues=stdatm(:,2)  SaturateOnIntegerOverflow=on
  p : Outport
  T : Outport  Port=2
  rho : Outport  Port=3
  a : Outport  Port=4
  wires:
  Saturation/1 -> Speed of sound  LUT/1, Density LUT/1, Pressure LUT/1, Temperature LUT/1
  Speed of sound  LUT/1 -> a/1
  Density LUT/1 -> rho/1
  Pressure LUT/1 -> p/1
  Temperature LUT/1 -> T/1
  MSLAlt/1 -> Saturation/1

== system aerosimlib/Atmosphere/Turbulence ==
  note: Sources
  note: Compute turbulence velocity and acceleration
  note: Outputs
  VelW : Inport  PortDimensions=[3 1]
  AGLAlt : Inport  Port=2  PortDimensions=1
  WindVel : Inport  Port=3  PortDimensions=[3 1]
  Demux1 : Demux  Outputs=3
  Lateral  Turbulence Filter : Subsystem  mask(Lateral turbulence filter){tsamp=tsamp}
      mask prompts: tsamp "Sample time [s]:"
      mask help: Shaping filter for lateral turbulence, using von Karman model.
  Longitudinal  Turbulence Filter : Subsystem  mask(Longitudinal turbulence filter){tsamp=tsamp}
      mask prompts: tsamp "Sample time [s]:"
      mask help: Shaping filter for longitudinal turbulence, using von Karman model.
  Mux : Mux  Inputs=3
  Mux1 : Mux  Inputs=3
  Terminator : Terminator
  Terminator1 : Terminator
  Turbulence Characteristics : Subsystem
      mask Type: Turbulence characteristics
      mask Description: Computes turbulence intensity and reference length as functions of altitude and background wind speed.
  Unit Delay : UnitDelay  X0=0.1  SampleTime=tsamp
  Vertical  Turbulence Filter : Subsystem  mask(Vertical turbulence filter){tsamp=tsamp}
      mask prompts: tsamp "Sample time [s]:"
      mask help: Shaping filter for vertical turbulence, using von Karman model.
  ft 2 m : aerosimlib/Unit Conversion/Distance/ft 2 m
  ft 2 m1 : aerosimlib/Unit Conversion/Distance/ft 2 m
  m 2 ft : aerosimlib/Unit Conversion/Distance/m 2 ft
  m 2 ft1 : aerosimlib/Unit Conversion/Distance/m 2 ft
  m 2 ft2 : aerosimlib/Unit Conversion/Distance/m 2 ft
  TurbVel : Outport
  TurbAcc : Outport  Port=2
  wires:
  Demux1/1 -> m 2 ft/1
  VelW/1 -> Unit Delay/1
  AGLAlt/1 -> m 2 ft1/1
  m 2 ft/1 -> Lateral  Turbulence Filter/1(Airspeed), Vertical  Turbulence Filter/1(Airspeed), Longitudinal  Turbulence Filter/1(Airspeed)
  m 2 ft1/1 -> Turbulence Characteristics/1(AGLAlt)
  WindVel/1 -> m 2 ft2/1
  m 2 ft2/1 -> Turbulence Characteristics/2(WindVel)
  Turbulence Characteristics/1(sigmau) -> Longitudinal  Turbulence Filter/3(Intensity)
  Turbulence Characteristics/2(sigmav) -> Lateral  Turbulence Filter/3(Intensity)
  Turbulence Characteristics/3(sigmaw) -> Vertical  Turbulence Filter/3(Intensity)
  Turbulence Characteristics/4(Lu) -> Longitudinal  Turbulence Filter/2(RefLength)
  Turbulence Characteristics/5(Lv) -> Lateral  Turbulence Filter/2(RefLength)
  Turbulence Characteristics/6(Lw) -> Vertical  Turbulence Filter/2(RefLength)
  Longitudinal  Turbulence Filter/1(LongVel) -> Mux/1
  Longitudinal  Turbulence Filter/2(LongAcc) -> Mux1/1
  Lateral  Turbulence Filter/1(LatVel) -> Mux/2
  Lateral  Turbulence Filter/2(LatAcc) -> Mux1/2
  Vertical  Turbulence Filter/1(VertVel) -> Mux/3
  Vertical  Turbulence Filter/2(VertAcc) -> Mux1/3
  Mux/1 -> ft 2 m/1
  Mux1/1 -> ft 2 m1/1
  ft 2 m/1 -> TurbVel/1
  ft 2 m1/1 -> TurbAcc/1
  Demux1/2 -> Terminator/1
  Demux1/3 -> Terminator1/1
  Unit Delay/1 -> Demux1/1

== system aerosimlib/Atmosphere/Wind Shear ==
  note: Transversal wind shear
  note: Time derivatives of wind speed
      | in body axes
  note: Body velocities
  note: Lateral wind shear
  note: Vertical wind shear
  WindAcc : Inport  PortDimensions=[3 1]
  TurbAcc : Inport  Port=2  PortDimensions=[3 1]
  Velocities : Inport  Port=3  PortDimensions=[3 1]
  Demux : Demux  Outputs=3
  Demux1 : Demux  Outputs=3
  Derivative : Derivative
  Mux : Mux  Inputs=3
  Mux1 : Mux  Inputs=3
  Product1 : Product  Inputs=*/  SaturateOnIntegerOverflow=on  InputSameDT=on
  Product2 : Product  Inputs=*/  SaturateOnIntegerOverflow=on  InputSameDT=on
  Product3 : Product  Inputs=*/  SaturateOnIntegerOverflow=on  InputSameDT=on
  Sum : Sum  Inputs=|++  SaturateOnIntegerOverflow=on  InputSameDT=on
  Terminator : Terminator
  Terminator1 : Terminator
  Terminator2 : Terminator
  Zero : Constant  Value=0
  Zero Offset : aerosimlib/Math/Zero Offset  tol=10^-6
  Zero Offset1 : Subsystem  mask(Zero offset){tol=10^-6}
      mask prompts: tol "Tolerance"
      mask help: This block outputs a value equal to the tolerance specified in the block parameters if the input falls within a sphere with this tolerance as radius and center in the origin. Otherwise, the output equals the input.
  Zero Offset2 : Subsystem  mask(Zero offset){tol=10^-6}
      mask prompts: tol "Tolerance"
      mask help: This block outputs a value equal to the tolerance specified in the block parameters if the input falls within a sphere with this tolerance as radius and center in the origin. Otherwise, the output equals the input.
  WindAngRates : Outport
  WindAngAcc : Outport  Port=2
  wires:
  Product3/1 -> Terminator2/1
  Mux1/1 -> Derivative/1
  Zero Offset2/1(Out) -> Product1/2
  Zero Offset1/1(Out) -> Product2/2
  Derivative/1 -> WindAngAcc/1
  Sum/1 -> Demux1/1
  TurbAcc/1 -> Sum/2
  WindAcc/1 -> Sum/1
  Mux/1 -> WindAngRates/1
  Zero/1 -> Mux/1, Mux1/1, Mux1/3, Mux1/2
  Demux1/2 -> Product2/1
  Demux1/3 -> Product1/1, Product3/1
  Demux1/1 -> Terminator/1
  Velocities/1 -> Demux/1
  Demux/1 -> Zero Offset2/1(In), Zero Offset1/1(In)
  Demux/2 -> Zero Offset/1
  Demux/3 -> Terminator1/1
  Product1/1 -> Mux/2
  Product2/1 -> Mux/3
  Zero Offset/1 -> Product3/2
